simulink model "am_sys"  (Simulink 3.00)
settings: Solver=ode45  StartTime=0.0  StopTime=999999  MaxStep=0.001  RelTol=1e-3  AbsTol=1e-3
undefined symbols (not defined in the file): at, bt, ct, dt
settings Model: SaveTime=off  SaveOutput=off

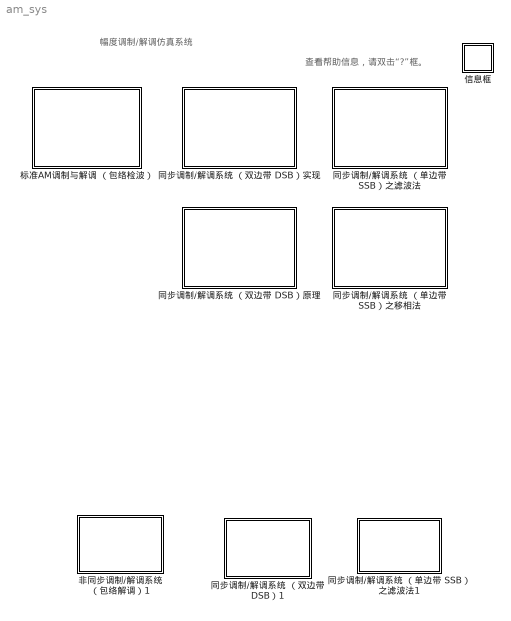
== system am_sys ==
  note: 幅度调制/解调仿真系统
  note: 查看帮助信息，请双击“?”框。
  标准AM调制与解调 （包络检波） : Subsystem
      settings: OpenFcn=am_sys1
      mask Display: disp('Standard\nAM System')
  非同步调制/解调系统 （包络解调）1 : Subsystem
      mask Display: disp('AM\nSystem - 1')
  同步调制/解调系统 （单边带 SSB） 之滤波法1 : Subsystem
      mask Display: disp('AM\nSystem - 3')
  同步调制/解调系统 （单边带 SSB）之滤波法 : Subsystem
      settings: OpenFcn=am_sys3
      mask Display: disp('AM - SSB\n（滤波法）')
  同步调制/解调系统 （单边带 SSB）之移相法 : Subsystem
      settings: OpenFcn=am_sys4
      mask Display: disp('AM - SSB\n（移相法）')
  同步调制/解调系统 （双边带 DSB）1 : Subsystem
      mask Display: disp('AM\nSystem - 2')
  同步调制/解调系统 （双边带 DSB）实现 : Subsystem
      settings: OpenFcn=am_sys2
      mask Display: disp('AM - DSB\n（实现）')
  同步调制/解调系统 （双边带 DSB）原理 : Subsystem
      settings: OpenFcn=am_sys5
      mask Display: disp('AM - DSB\n（原理）')
  信息框 : Subsystem
      mask Display: disp('?')

== system am_sys/标准AM调制与解调 （包络检波） ==

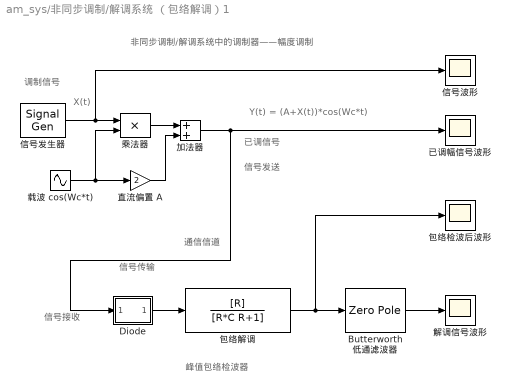
== system am_sys/非同步调制/解调系统 （包络解调）1 ==
  note: 非同步调制/解调系统中的调制器——幅度调制
  note: 信号接收
  note: 信号传输
  note: 通信信道
  note: 信号发送
  note: 已调信号
  note: Y(t) = (A+X(t))*cos(Wc*t)
  note: X(t)
  note: 调制信号
  note: 峰值包络检波器
  Butterworth 低通滤波器 : ZeroPole  Zeros=z  Poles=p  Gain=k  mask(buttap){@1=5*2*pi, @2=4}
      mask prompts: @1 "Cutoff frequency (rad/sec)"; @2 "Order"
      mask help:
      | Analog Butterworth low pass filter.
      |
      | (Requires Signal Processing Toolbox)
      mask init:
      | [z,p,k]=buttap(@2); z=@1*z; p=@1*p; k=real(prod(-p)); [num,den]=zp2tf(z,p,k); w=logspace(log10(@1/10),log10(10*@1),20); h=freqs(num,den,w);
      mask Help: Butterworth low pass filter using MATLAB's butter command.
      mask Display: plot(20*log10(w),20*log10(abs(h)))
  Diode : Subsystem
      mask Type: 二极管
      mask Description: 二极管
      mask Display: plot([0 2 2 2],[0 0 2 -2],[2 4],[2 0],[2 4],[-2 0],[4 4 4 6],[-2 2 0 0]);
  包络检波后波形 : Scope
      settings: TimeRange=1.000000  YMin=-1.000000  YMax=1.000000  SaveToWorkspace=off  SaveName=ScopeData  DataFormat=Matrix
  包络解调 : TransferFcn  Numerator=[R]  Denominator=[R*C R+1]  mask(单元6){@1=1, @2=0.1}
      mask prompts: @1 "电阻值（欧）："; @2 "电容值（法）："
      mask help: 单元6
      mask init:
      | R=@1;C=@2;
      mask Display: plot([0 15],[2 2],[8 8 6 10],[2 0 0 0],[6 10],[-1 -1],[8 8 7 9],[-1 -4 -4 -4],[12.5 12.5 12 13],[2 1 1 1],[12 12],[1 -3],[13 13],[1 -3],[12 13 12.5 12.5],[-3 -3 -3 -4],[12 13],[-4 -4]);
  乘法器 : Product  Inputs=2  SaturateOnIntegerOverflow=on
      mask Type: 乘法器
      mask Description: 乘法器
      mask Display: plot([0 1],[1 0],[0 1],[0 1]);
  加法器 : Sum  Inputs=++  SaturateOnIntegerOverflow=on
  解调信号波形 : Scope
      settings: TimeRange=1.000000  YMin=-0.500000  YMax=0.500000  SaveToWorkspace=off  SaveName=ScopeData  DataFormat=Matrix
  信号波形 : Scope
      settings: TimeRange=1.000000  YMin=-3.000000  YMax=3.000000  SaveToWorkspace=off  SaveName=ScopeData  DataFormat=Matrix
  信号发生器 : SignalGenerator  WaveForm=sine  Amplitude=1.000000  Frequency=30.000000  Units=rad/sec
  已调幅信号波形 : Scope
      settings: TimeRange=1.000000  YMin=-3.000000  YMax=3.000000  SaveToWorkspace=off  SaveName=ScopeData  DataFormat=Matrix
  载波 cos(Wc*t) : Sin  Amplitude=1  Frequency=F*2*pi  Phase=0  SampleTime=-1  mask(载波){@1=50}
      mask prompts: @1 "载波频率（Hz）："
      mask help: 载波
      mask init:
      | F=@1;
  直流偏置 A : Gain  Gain=2  SaturateOnIntegerOverflow=on
  wires:
  包络解调/1 -> Butterworth 低通滤波器/1, 包络检波后波形/1
  乘法器/1 -> 加法器/1
  载波 cos(Wc*t)/1 -> 乘法器/2, 直流偏置 A/1
  直流偏置 A/1 -> 加法器/2
  加法器/1 -> 已调幅信号波形/1, Diode/1(in_1)
  Diode/1(out_1) -> 包络解调/1
  信号发生器/1 -> 乘法器/1, 信号波形/1
  Butterworth 低通滤波器/1 -> 解调信号波形/1

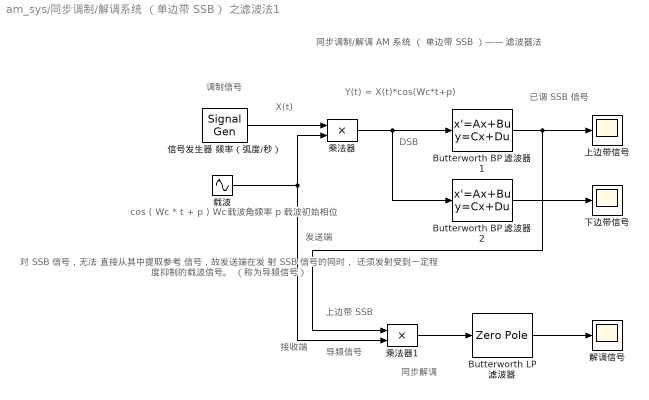
== system am_sys/同步调制/解调系统 （单边带 SSB） 之滤波法1 ==
  note: 接收端
  note: 发送端
  note: 对 SSB 信号，无法
      | 直接从其中提取参考
      | 信号，故发送端在发
      | 射 SSB 信号的同时，
      | 还须发射受到一定程
      | 度抑制的载波信号。
      | （称为导频信号）
  note: 已调 SSB 信号
  note: Y(t) = X(t)*cos(Wc*t+p)
  note: X(t)
  note: 调制信号
  note: cos ( Wc * t + p )
      | Wc 载波角频率
      | p 载波初始相位
  note: DSB
  note: 导频信号
  note: 上边带 SSB
  note: 同步调制/解调 AM 系统 （ 单边带 SSB ）—— 滤波器法
  note: 同步解调
  Butterworth BP 滤波器 1 : StateSpace  A=at  B=bt  C=ct  D=dt  X0=0  mask(buttap,lp2bp){@1=110, @2=5, @3=4}
      mask prompts: @1 "Center frequency (rad/sec)"; @2 "Bandwidth (rad/sec):"; @3 "Order"
      mask help:
      | Analog Butterworth band pass filter.
      |
      | (Requires Signal Processing Toolbox)
      mask init:
      | [at,bt,ct,dt,w,mag]=filtm('buttap','lp2bp',@1,@2,50,@3);
      mask Help: Butterworth band pass filter using MATLAB's butter and lp2bp command.
      mask Display: plot(w,mag)
  Butterworth BP 滤波器 2 : StateSpace  A=at  B=bt  C=ct  D=dt  X0=0  mask(buttap,lp2bp){@1=90, @2=5, @3=4}
      mask prompts: @1 "Center frequency (rad/sec)"; @2 "Bandwidth (rad/sec):"; @3 "Order"
      mask help:
      | Analog Butterworth band pass filter.
      |
      | (Requires Signal Processing Toolbox)
      mask init:
      | [at,bt,ct,dt,w,mag]=filtm('buttap','lp2bp',@1,@2,50,@3);
      mask Help: Butterworth band pass filter using MATLAB's butter and lp2bp command.
      mask Display: plot(w,mag)
  Butterworth LP 滤波器 : ZeroPole  Zeros=z  Poles=p  Gain=k  mask(buttap){@1=15, @2=4}
      mask prompts: @1 "Cutoff frequency (rad/sec)"; @2 "Order"
      mask help:
      | Analog Butterworth low pass filter.
      |
      | (Requires Signal Processing Toolbox)
      mask init:
      | [z,p,k]=buttap(@2); z=@1*z; p=@1*p; k=real(prod(-p)); [num,den]=zp2tf(z,p,k); w=logspace(log10(@1/10),log10(10*@1),20); h=freqs(num,den,w);
      mask Help: Butterworth low pass filter using MATLAB's butter command.
      mask Display: plot(20*log10(w),20*log10(abs(h)))
  乘法器 : Product  Inputs=2  SaturateOnIntegerOverflow=on
      mask Type: 乘法器
      mask Description: 乘法器
      mask Display: plot([0 1],[1 0],[0 1],[0 1]);
  乘法器1 : Product  Inputs=2  SaturateOnIntegerOverflow=on
      mask Type: 乘法器
      mask Description: 乘法器
      mask Display: plot([0 1],[1 0],[0 1],[0 1]);
  解调信号 : Scope
      settings: TimeRange=1.000000  YMin=-1.000000  YMax=1.000000  SaveToWorkspace=off  SaveName=ScopeData  DataFormat=Matrix
  上边带信号 : Scope
      settings: TimeRange=1.000000  YMin=-2.000000  YMax=2.000000  SaveToWorkspace=off  SaveName=ScopeData  DataFormat=Matrix
  下边带信号 : Scope
      settings: TimeRange=1.000000  YMin=-2.000000  YMax=2.000000  SaveToWorkspace=off  SaveName=ScopeData  DataFormat=Matrix
  信号发生器 频率（弧度/秒） : SignalGenerator  WaveForm=sine  Amplitude=1.000000  Frequency=10.000000  Units=rad/sec
  载波 : Sin  Amplitude=1  Frequency=100  Phase=0  SampleTime=-1
  wires:
  信号发生器 频率（弧度/秒）/1 -> 乘法器/1
  乘法器/1 -> Butterworth BP 滤波器 1/1, Butterworth BP 滤波器 2/1
  Butterworth BP 滤波器 2/1 -> 下边带信号/1
  载波/1 -> 乘法器/2, 乘法器1/2
  Butterworth BP 滤波器 1/1 -> 上边带信号/1, 乘法器1/1
  乘法器1/1 -> Butterworth LP 滤波器/1
  Butterworth LP 滤波器/1 -> 解调信号/1

== system am_sys/同步调制/解调系统 （单边带 SSB）之滤波法 ==

== system am_sys/同步调制/解调系统 （单边带 SSB）之移相法 ==

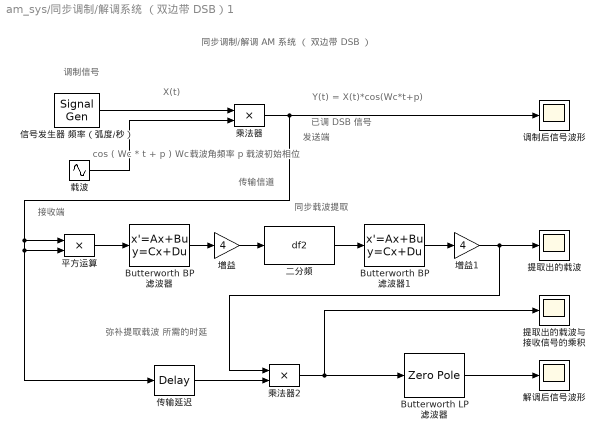
== system am_sys/同步调制/解调系统 （双边带 DSB）1 ==
  note: 传输信道
  note: cos ( Wc * t + p )
      | Wc 载波角频率
      | p 载波初始相位
  note: 同步调制/解调 AM 系统 （ 双边带 DSB ）
  note: 同步载波提取
  note: 接收端
  note: 已调 DSB 信号
  note: 发送端
  note: Y(t) = X(t)*cos(Wc*t+p)
  note: X(t)
  note: 调制信号
  note: 弥补提取载波
      | 所需的时延
  Butterworth BP 滤波器 : StateSpace  A=at  B=bt  C=ct  D=dt  X0=0  mask(buttap,lp2bp){@1=200, @2=10, @3=4}
      mask prompts: @1 "Center frequency (rad/sec)"; @2 "Bandwidth (rad/sec):"; @3 "Order"
      mask help:
      | Analog Butterworth band pass filter.
      |
      | (Requires Signal Processing Toolbox)
      mask init:
      | [at,bt,ct,dt,w,mag]=filtm('buttap','lp2bp',@1,@2,50,@3);
      mask Help: Butterworth band pass filter using MATLAB's butter and lp2bp command.
      mask Display: plot(w,mag)
  Butterworth BP 滤波器1 : StateSpace  A=at  B=bt  C=ct  D=dt  X0=0  mask(buttap,lp2bp){@1=100, @2=10, @3=4}
      mask prompts: @1 "Center frequency (rad/sec)"; @2 "Bandwidth (rad/sec):"; @3 "Order"
      mask help:
      | Analog Butterworth band pass filter.
      |
      | (Requires Signal Processing Toolbox)
      mask init:
      | [at,bt,ct,dt,w,mag]=filtm('buttap','lp2bp',@1,@2,50,@3);
      mask Help: Butterworth band pass filter using MATLAB's butter and lp2bp command.
      mask Display: plot(w,mag)
  Butterworth LP 滤波器 : ZeroPole  Zeros=z  Poles=p  Gain=k  mask(buttap){@1=10, @2=4}
      mask prompts: @1 "Cutoff frequency (rad/sec)"; @2 "Order"
      mask help:
      | Analog Butterworth low pass filter.
      |
      | (Requires Signal Processing Toolbox)
      mask init:
      | [z,p,k]=buttap(@2); z=@1*z; p=@1*p; k=real(prod(-p)); [num,den]=zp2tf(z,p,k); w=logspace(log10(@1/10),log10(10*@1),20); h=freqs(num,den,w);
      mask Help: Butterworth low pass filter using MATLAB's butter command.
      mask Display: plot(20*log10(w),20*log10(abs(h)))
  乘法器 : Product  Inputs=2  SaturateOnIntegerOverflow=on
      mask Type: 乘法器
      mask Description: 乘法器
      mask Display: plot([0 1],[1 0],[0 1],[0 1]);
  乘法器2 : Product  Inputs=2  SaturateOnIntegerOverflow=on
      mask Type: 乘法器
      mask Description: 乘法器
      mask Display: plot([0 1],[1 0],[0 1],[0 1]);
  传输延迟 : TransportDelay  DelayTime=0.09  InitialInput=0  BufferSize=1024
  调制后信号波形 : Scope
      settings: TimeRange=1.000000  YMin=-2.000000  YMax=2.000000  SaveToWorkspace=off  SaveName=ScopeData  DataFormat=Matrix
  二分频 : MATLABFcn  MATLABFcn=df2  OutputWidth=-1  OutputSignalType=auto
      mask Type: 分频器
      mask Description: 二分频器
      mask Display: disp('Frequency\n—————\n2')
  解调后信号波形 : Scope
      settings: TimeRange=1.000000  YMin=-2.000000  YMax=2.000000  SaveToWorkspace=off  SaveName=ScopeData  DataFormat=Matrix
  平方运算 : Product  Inputs=2  SaturateOnIntegerOverflow=on
      mask Type: 乘法器
      mask Description: 乘法器
      mask Display: plot([0 1],[1 0],[0 1],[0 1]);
  提取出的载波 : Scope
      settings: TimeRange=1.000000  YMin=-4.000000  YMax=4.000000  SaveToWorkspace=off  SaveName=ScopeData  DataFormat=Matrix
  提取出的载波与 接收信号的乘积 : Scope
      settings: TimeRange=1.000000  YMin=-4.000000  YMax=4.000000  SaveToWorkspace=off  SaveName=ScopeData  DataFormat=Matrix
  信号发生器 频率（弧度/秒） : SignalGenerator  WaveForm=sine  Amplitude=1.000000  Frequency=10.000000  Units=rad/sec
  载波 : Sin  Amplitude=1  Frequency=100  Phase=0  SampleTime=-1
  增益 : Gain  Gain=4  SaturateOnIntegerOverflow=on
  增益1 : Gain  Gain=4  SaturateOnIntegerOverflow=on
  wires:
  乘法器/1 -> 调制后信号波形/1, 平方运算/1, 传输延迟/1, 平方运算/2
  乘法器2/1 -> Butterworth LP 滤波器/1, 提取出的载波与 接收信号的乘积/1
  Butterworth LP 滤波器/1 -> 解调后信号波形/1
  增益1/1 -> 提取出的载波/1, 乘法器2/1
  传输延迟/1 -> 乘法器2/2
  Butterworth BP 滤波器1/1 -> 增益1/1
  二分频/1 -> Butterworth BP 滤波器1/1
  增益/1 -> 二分频/1
  Butterworth BP 滤波器/1 -> 增益/1
  平方运算/1 -> Butterworth BP 滤波器/1
  载波/1 -> 乘法器/2
  信号发生器 频率（弧度/秒）/1 -> 乘法器/1

== system am_sys/同步调制/解调系统 （双边带 DSB）实现 ==

== system am_sys/同步调制/解调系统 （双边带 DSB）原理 ==

== system am_sys/信息框 ==
  note: 窗口中每一个框图代表着一个完整的 AM 系统，包括信息的发送端和接收端模块仿真，
  note: 幅度调制/解调仿真系统
  note: 2。同步调制/解调 AM 系统（双边带 DSB）
  note: 3。同步调制/解调 AM 系统（单边带 SSB）
  note: 系利用 MATLAB 中的 SIMULINK 板块制作。
  note: 以及连接两端的信道（用一信号连线表示）。窗口中包括如下几个独立的 AM 系统：
  note: 用鼠标指向要查看的系统方框，然后在其上双击即可。
  note: 1。非同步调制/解调 AM 系统（包络检波）

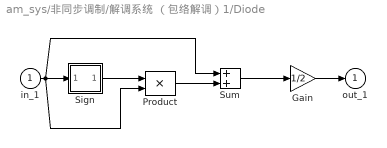
== system am_sys/非同步调制/解调系统 （包络解调）1/Diode ==
  in_1 : Inport  Port=1  PortWidth=-1  SampleTime=-1  DataType=auto
      settings: SignalType=auto
  Gain : Gain  Gain=1/2  SaturateOnIntegerOverflow=on
  Product : Product  Inputs=2  SaturateOnIntegerOverflow=on
  Sign : Subsystem
      mask Type: Sign
      mask Description: y = sign(x)
      mask Help: Sign Function:\n\t\t\ty = 1 if x > 0\n\t\t\ty = 0 if x = 0\n\t\t\ty = -1 if x < 0
      mask Display: plot(-50,-50,50,50,[-50,50],[0,0],[0,0],[-50,50],[-40,0],[-30,-30],[0,40],[30,30])
  Sum : Sum  Inputs=++  SaturateOnIntegerOverflow=on
  out_1 : Outport  Port=1
  wires:
  Gain/1 -> out_1/1
  Sign/1(out_1) -> Product/1
  in_1/1 -> Sign/1(in_1), Product/2, Sum/1
  Product/1 -> Sum/2
  Sum/1 -> Gain/1

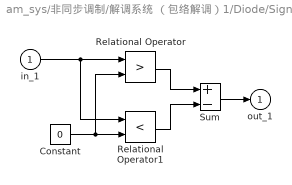
== system am_sys/非同步调制/解调系统 （包络解调）1/Diode/Sign ==
  in_1 : Inport  Port=1  PortWidth=-1  SampleTime=-1  DataType=auto
      settings: SignalType=auto
  Constant : Constant  Value=0
  Relational Operator : RelationalOperator  Operator=>
  Relational Operator1 : RelationalOperator  Operator=<
  Sum : Sum  Inputs=+-  SaturateOnIntegerOverflow=on
  out_1 : Outport  Port=1
  wires:
  Sum/1 -> out_1/1
  Relational Operator/1 -> Sum/1
  Relational Operator1/1 -> Sum/2
  Constant/1 -> Relational Operator1/2, Relational Operator/2
  in_1/1 -> Relational Operator/1, Relational Operator1/1
